simulink model "electric_motor"  (R2016b)
settings: Solver=VariableStepAuto  StartTime=0.0  StopTime=10.0  RelTol=1e-3
values from neighbouring files (symbols this model uses):
  b = 0.019029892    [inertia_estimation.mat]    (also in motor_parameters.mat)
  beta = 0.001610902    [inertia_estimation.mat]    (also in motor_parameters.mat)
  J = 0.00123078313678    [inertia_estimation.mat]    (also in motor_parameters.mat)
  m = abs(matrix - diag(diag(matrix)))    [is_diagonal.m]
  R = 2.4    [inertia_estimation.mat]    (also in motor_parameters.mat)
undefined symbols (not defined in the file): K_e, K_t
libraries: nesl_utility x5, sm_lib x4, simulink x1
settings Model: Creator=piotr  LastModifiedBy=piotr

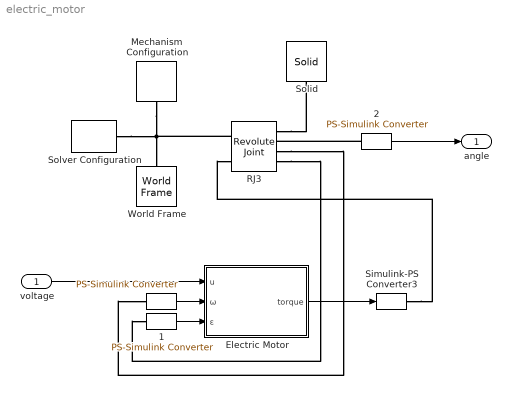
== system electric_motor ==
  voltage : Inport
  "  " : nesl_utility/PS-Simulink Converter  PhysicalDomain=network_engine_domain  SubClassName=ps_output  LeftPortType=input  RightPortType=output  PseudoPeriodic=off  Frequencies=[]  Unit=1  AffineConversion=off
  "  1" : nesl_utility/PS-Simulink Converter  PhysicalDomain=network_engine_domain  SubClassName=ps_output  LeftPortType=input  RightPortType=output  PseudoPeriodic=off  Frequencies=[]  Unit=1  AffineConversion=off
  " 2" : nesl_utility/PS-Simulink Converter  PhysicalDomain=network_engine_domain  SubClassName=ps_output  LeftPortType=input  RightPortType=output  PseudoPeriodic=off  Frequencies=[]  Unit=1  AffineConversion=off
  Electric Motor : Subsystem  mask{k_e=K_e, k_t=K_t, R=R, beta=beta, b=b, J=J, k_gear=1}
      mask prompts: k_e "Electromotive force constant [V*s/rad]"; k_t "Motor torque constant [N*m/A]"; R "Electrical resistance [Ω]"; beta "Motor viscous damping [N*m*s/rad]"; b "Motor dry damping [N*m]"; J "Motor moment of inertia [kg*m^2]"; k_gear "Gearbox constant"
  Mechanism Configuration : sm_lib/Utilities/Mechanism Configuration  UniformGravity=Constant  GravityVector=[0 0 -9.80665]  GravityUnits=m/s^2  LinearizationDelta=0.001
  RJ3 : sm_lib/Joints/Revolute Joint  SenseConstraintForce=off  SenseConstraintForceX=off  SenseConstraintForceY=off  SenseConstraintForceZ=off  SenseConstraintTorque=off  SenseConstraintTorqueX=off  SenseConstraintTorqueY=off  SenseConstraintTorqueZ=off  SenseTotalForce=off  SenseTotalForceX=off  SenseTotalForceY=off  SenseTotalForceZ=off  SenseTotalTorque=off  SenseTotalTorqueX=off  SenseTotalTorqueY=off  SenseTotalTorqueZ=off  CompositeWrenchDir=FollowerOnBase  CompositeWrenchFrame=BaseFrame  EquilibriumPosition=0  EquilibriumPositionUnits=rad  SpringStiffness=0  SpringStiffnessUnits=N*m/deg  DampingCoefficient=0  DampingCoefficientUnits=N*m/(deg/s)  TorqueActuationMode=InputTorque  MotionActuationMode=ComputedMotion  SensePosition=on  SenseVelocity=on  SenseAcceleration=on  SenseTorqueForce=off  PositionTargetSpecify=off  PositionTargetPriority=Low  PositionTargetValue=0.5*pi  PositionTargetValueUnits=rad  VelocityTargetSpecify=off  VelocityTargetPriority=Low  VelocityTargetValue=0  VelocityTargetValueUnits=rad/s
  Simulink-PS Converter3 : nesl_utility/Simulink-PS Converter  PhysicalDomain=network_engine_domain  SubClassName=ps_input  LeftPortType=input  RightPortType=output  PseudoPeriodic=off  Frequencies=[]  NoiseDistribution=none  NoiseParameters=[]  Unit=N*m  AffineConversion=off  InputFiltering=off  SimscapeFilterOrder=1  InputFilterTimeConstant=.001  UdotUserProvided=1
  Solid : sm_lib/Body Elements/Solid  InertiaType=CalculateFromGeometry  Mass=0.001  MassUnits=g  CenterOfMass=[0 0 0]  CenterOfMassUnits=m  MomentsOfInertia=[1 1 1]  MomentsOfInertiaUnits=kg*m^2  ProductsOfInertia=[1 1 1]  ProductsOfInertiaUnits=kg*m^2  DensityBased=off  Density=1000  DensityUnits=kg/m^3  DoExposeReferenceFrame=on  SerializedFrames=<Frames/>  GraphicType=FromGeometry  MarkerShape=Sphere  MarkerSize=10  GraphicVisPropType=SimpleVisualProperties  GraphicDiffuseColor=[0.5 0.5 0.5]  GraphicSpecularColor=[0.5 0.5 0.5 1.0]  GraphicAmbientColor=[0.15 0.15 0.15 1.0]  GraphicEmissiveColor=[0.0 0.0 0.0 1.0]  GraphicShininess=75  GraphicOpacity=1.0  GeometryShape=Brick  RectangleSize=[1 1]  RectangleSizeUnits=m  BrickDimensions=[1 1 1]  BrickDimensionUnits=cm  CylinderRadius=1  CylinderRadiusUnits=m  CylinderLength=1  CylinderLengthUnits=m  SphereRadius=1  SphereRadiusUnits=m  EllipsoidRadii=[1 1 1]  EllipsoidRadiiUnits=m  ExtrusionCrossSection=[1 1; -1 1; -1 -1; 1 -1]  ExtrusionCrossSectionUnits=m  ExtrusionLength=1  ExtrusionLengthUnits=m  PolygonNumSides=3  PolygonOuterRadius=1  PolygonOuterRadiusUnits=m  ExtGeomFileType=STEP  ExtGeomFileUnits=m  RevolutionCrossSection=[1 1; 1 -1; 2 -1; 2 1]  RevolutionCrossSectionUnits=m  RevolutionExtent=Full  RevolutionAngle=180  RevolutionAngleUnits=deg
  Solver Configuration : nesl_utility/Solver Configuration  PhysicalDomain=network_engine_domain  SubClassName=solver  LeftPortType=input  RightPortType=generic  Accelerate=off  Tones=[]  Harmonics=[]  SimulateNoise=off  Profile=off  UseLocalSampling=off  EnableSwitchedLinearOptims=on  FrequencyDomain=off  UseCCode=off  RelTol=0.001  AbsTol=1e-06  MinStep=1e-09  ToWorkspace=off  RevertToSquareIcSolve=off  NumHomotopyIterations=100  PhasorMode=off  PhasorModeNumHarmonics=1  OverrideAbsTol=off  DoDC=off  ResidualTolerance=1e-09  UseLocalSolver=off  LocalSolverChoice=NE_BACKWARD_EULER_ADVANCER  LocalSolverSampleTime=0.001  DoFixedCost=off  MaxNonlinIter=3  MaxModeIter=2  LinearAlgebra=Sparse  DelaysMemoryBudget=1024  AutomaticFiltering=on  FilteringTimeConstant=0.001
  World Frame : sm_lib/Frames and Transforms/World Frame
  angle : Outport
  wires:
  "  "/1 -> Electric Motor/2(ω)
  "  1"/1 -> Electric Motor/3(ε)
  Electric Motor/1(torque) -> Simulink-PS Converter3/1
  voltage/1 -> Electric Motor/1(u)
  " 2"/1 -> angle/1
  connections:
  Solver Configuration/RConn1 -- RJ3/LConn1 -- Mechanism Configuration/RConn1 -- World Frame/RConn1
  Simulink-PS Converter3/RConn1 -- RJ3/LConn2
  RJ3/RConn4 -- "  1"/LConn1
  RJ3/RConn3 -- "  "/LConn1
  " 2"/LConn1 -- RJ3/RConn2
  RJ3/RConn1 -- Solid/RConn1

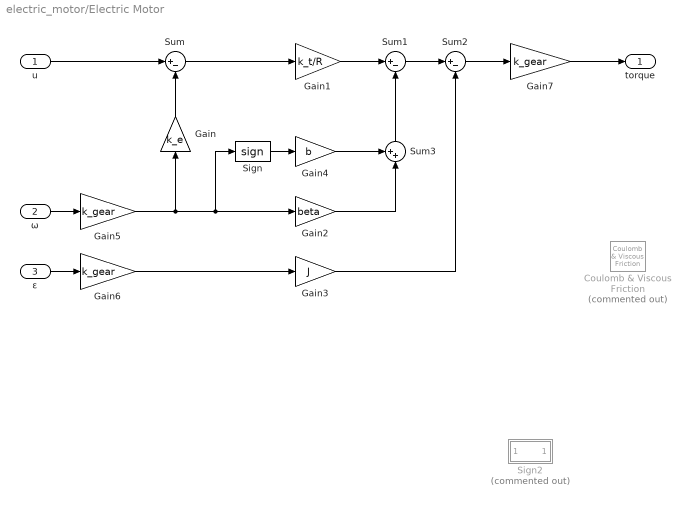
== system electric_motor/Electric Motor ==
  u : Inport
  ω : Inport  Port=2
  ε : Inport  Port=3
  Coulomb & Viscous Friction : simulink/Discontinuities/Coulomb & Viscous Friction  Commented=on  offset=[1 3 2 0]  gain=1
  Gain : Gain  Gain=k_e
  Gain1 : Gain  Gain=k_t/R
  Gain2 : Gain  Gain=beta
  Gain3 : Gain  Gain=J
  Gain4 : Gain  Gain=b
  Gain5 : Gain  Gain=k_gear
  Gain6 : Gain  Gain=k_gear
  Gain7 : Gain  Gain=k_gear
  Sign : Signum  ZeroCross=off
  Sign2 : Subsystem  Commented=on
  Sum : Sum  Inputs=|+-
  Sum1 : Sum  Inputs=|+-
  Sum2 : Sum  Inputs=|+-
  Sum3 : Sum  Inputs=++|
  torque : Outport
  wires:
  Sum/1 -> Gain1/1
  Gain/1 -> Sum/2
  ω/1 -> Gain5/1
  Gain1/1 -> Sum1/1
  Sum1/1 -> Sum2/1
  Sum2/1 -> Gain7/1
  Gain3/1 -> Sum2/2
  ε/1 -> Gain6/1
  u/1 -> Sum/1
  Gain5/1 -> Sign/1, Gain2/1, Gain/1
  Gain6/1 -> Gain3/1
  Gain7/1 -> torque/1
  Sign/1 -> Gain4/1
  Gain4/1 -> Sum3/1
  Gain2/1 -> Sum3/2
  Sum3/1 -> Sum1/2

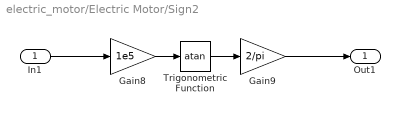
== system electric_motor/Electric Motor/Sign2 ==
  In1 : Inport
  Gain8 : Gain  Gain=1e5
  Gain9 : Gain  Gain=2/pi
  Trigonometric Function : Trigonometry  Operator=atan
  Out1 : Outport
  wires:
  Trigonometric Function/1 -> Gain9/1
  Gain8/1 -> Trigonometric Function/1
  Gain9/1 -> Out1/1
  In1/1 -> Gain8/1
